simulink model "Aufgabe4_wirkungsplan"  (Simulink 9.2)
settings: Solver=VariableStepAuto  StartTime=0.0  StopTime=10.0  RelTol=1e-3
settings Model: Creator=danial  LastModifiedBy=danial
settings DataIOCC: LimitDataPoints=off  SaveFormat=Dataset  SignalLoggingSaveFormat=Dataset
settings OptimizationCC: LifeSpan=auto
settings DebuggingCC: UnderspecifiedInitializationDetection=Simplified  MergeDetectMultiDrivingBlocksExec=error  FcnCallInpInsideContextMsg=error  StateNameClashWarn=none  SFUnexpectedBacktrackingDiag=error  SFNoUnconditionalDefaultTransitionDiag=error  SFExecutionAtInitializationDiag=warning
settings HardwareCC: ProdBitPerPointer=64  ProdBitPerSizeT=64  ProdBitPerPtrDiffT=64  ProdLargestAtomicFloat=Float  ProdIntDivRoundTo=Zero  ProdEndianess=LittleEndian  ProdWordSize=64  ProdHWDeviceType=Intel->x86-64 (Windows64)
settings ModelReferenceCC: PropagateSignalLabelsOutOfModel=on
settings CodeAppCC: StateflowObjectComments=off
settings GRTTargetCC: TargetLangStandard=C99 (ISO)  GeneratePreprocessorConditionals=Use local settings  CombineOutputUpdateFcns=on  GRTInterface=off
settings ConfigComp: CovMetricSettings=dwe  CovHtmlReporting=off  CovSaveCumulativeToWorkspaceVar=off  CovSaveSingleToWorkspaceVar=off  CovExternalEMLEnable=on

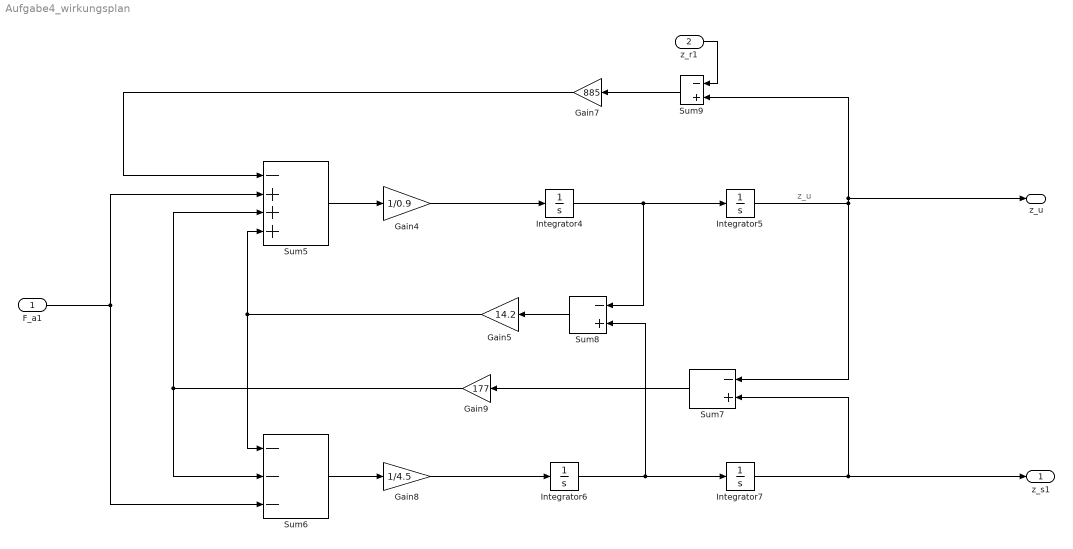
== system Aufgabe4_wirkungsplan ==
  note: z_u
  F_a1 : Inport  PortDimensions=1
  z_r1 : Inport  Port=2  PortDimensions=1
  Gain4 : Gain  Gain=1/0.9
  Gain5 : Gain  Gain=14.2
  Gain7 : Gain  Gain=885
  Gain8 : Gain  Gain=1/4.5
  Gain9 : Gain  Gain=177
  Integrator{4..7} (4 alike) : Integrator
  Sum5 : Sum  Inputs=-+++
  Sum6 : Sum  Inputs=---
  Sum7 : Sum  Inputs=-+
  Sum8 : Sum  Inputs=-+
  Sum9 : Sum  Inputs=-+
  z_s1 : Outport  PortDimensions=1
  z_u : Outport  Port=2  PortDimensions=1
  wires:
  F_a1/1 -> Sum6/3, Sum5/2
  Sum6/1 -> Gain8/1
  z_r1/1 -> Sum9/1
  Sum8/1 -> Gain5/1
  Sum5/1 -> Gain4/1
  Gain5/1 -> Sum5/4, Sum6/1
  Integrator5/1 -> Sum9/2, z_u/1, Sum7/1
  Sum7/1 -> Gain9/1
  Gain9/1 -> Sum5/3, Sum6/2
  Gain7/1 -> Sum5/1
  Sum9/1 -> Gain7/1
  Gain4/1 -> Integrator4/1
  Integrator6/1 -> Integrator7/1, Sum8/2
  Integrator4/1 -> Sum8/1, Integrator5/1
  Integrator7/1 -> z_s1/1, Sum7/2
  Gain8/1 -> Integrator6/1
